simulink model "MotorIdentVel"  (R2013a)
settings: Solver=FixedStepDiscrete  StartTime=0.0  StopTime=Time  FixedStep=0.01  RelTol=1e-3
values from neighbouring files (symbols this model uses):
  joint = CoupledJoints('experiments', 'iCubGenova03', 'torso')    [CoupledExper-IDLE.m]    (also in CoupledExper.m = joint.loadRefFile('ref'); CoupledJoints.m = [joint Motor(date,robotName, part, type,'yaw')]; FrictionTest.m = joint.loadFriction('idle.mat',1); JointStructure.m = struct)
undefined symbols (not defined in the file): Time
libraries: simulink x8, WBCLibrary x7, utility x1
settings Model: Creator=Raffaello  LastModifiedBy=Raffaello
settings DataIOCC: LimitDataPoints=off  OutputSaveName=out

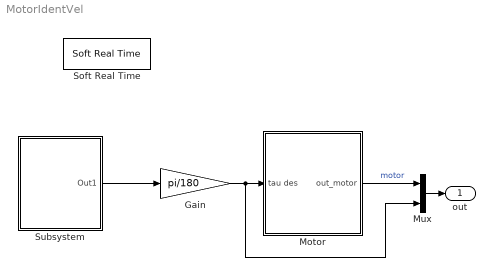
== system MotorIdentVel ==
  Gain : Gain  Gain=pi/180
  Motor : Subsystem
  Mux : Mux  Inputs=2
  Soft Real Time : utility/Soft Real Time  x=1
  Subsystem : Subsystem  mask{time_max=2, time=Time, K=10}
      mask prompts: time_max "Time to max"; K "Max value"
  out : Outport
  wires:
  Motor/1(out_motor) -> Mux/1  "motor"
  Mux/1 -> out/1
  Gain/1 -> Mux/2, Motor/1(tau des)
  Subsystem/1(Out1) -> Gain/1

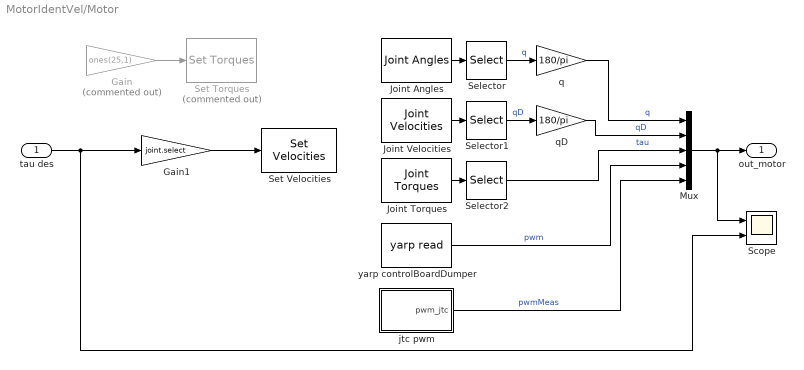
== system MotorIdentVel/Motor ==
  tau des : Inport
  Gain : Gain  Commented=on  Gain=ones(25,1)
  Gain1 : Gain  Gain=joint.select
  Joint Angles : WBCLibrary/wholeBodyStates/Joint Angles  robotName=robotName  localName=localName
  Joint Torques : WBCLibrary/wholeBodyStates/Joint Torques  robotName=robotName  localName=localName
  Joint Velocities : WBCLibrary/wholeBodyStates/Joint Velocities  robotName=robotName  localName=localName
  Mux : Mux  Inputs=5
  Scope : Scope  NumInputPorts=2
      settings: ShowLegends=on  TimeRange=10  YMin=-125~-2  YMax=125~1.5  SaveName=ScopeData2
  Selector : Selector  InputPortWidth=25  IndexOptions=Index vector (dialog)  Indices=[joint.number]  OutputSizes=1
  Selector1 : Selector  InputPortWidth=25  IndexOptions=Index vector (dialog)  Indices=[joint.number]  OutputSizes=1
  Selector2 : Selector  InputPortWidth=25  IndexOptions=Index vector (dialog)  Indices=[joint.number]  OutputSizes=1
  Set Torques : WBCLibrary/wholeBodyActuators/Set Torques  Commented=on  val=6  robotName=robotName  localName=localName
  Set Velocities : WBCLibrary/wholeBodyActuators/Set Velocities  val=4  robotName=robotName  localName=localName
  jtc pwm : Subsystem
  q : Gain  Gain=180/pi
  qD : Gain  Gain=180/pi
  yarp controlBoardDumper : WBCLibrary/Utilities/yarp read  from=['/controlBoardDumper/' joint.path '/getOutputs']  to='...'  num=1  blocking=off  timestamp=off
  out_motor : Outport
  wires:
  Gain/1 -> Set Torques/1
  Joint Velocities/1 -> Selector1/1
  Mux/1 -> out_motor/1, Scope/1
  Joint Angles/1 -> Selector/1
  Joint Torques/1 -> Selector2/1
  yarp controlBoardDumper/1 -> Mux/4  "pwm"
  Selector/1 -> q/1  "q"
  Selector1/1 -> qD/1  "qD"
  Selector2/1 -> Mux/3  "tau"
  q/1 -> Mux/1  "q"
  qD/1 -> Mux/2  "qD"
  jtc pwm/1(pwm_jtc) -> Mux/5  "pwmMeas"
  tau des/1 -> Gain1/1, Scope/2
  Gain1/1 -> Set Velocities/1

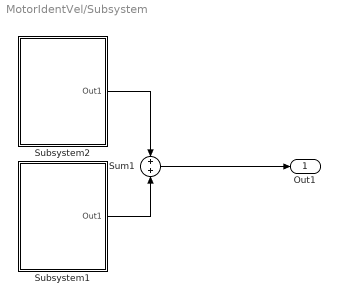
== system MotorIdentVel/Subsystem ==
  Subsystem1 : Subsystem  mask{time_max=time_max, init=0, K=-K, tot_time=time/2, time_start=time/2}
      mask prompts: time_max "Time to max"; init "Initial value"; K "Max value"; tot_time "Total time"; time_start "Time start"
  Subsystem2 : Subsystem  mask{time_max=time_max, init=0, K=K, tot_time=time/2, time_start=0}
      mask prompts: time_max "Time to max"; init "Initial value"; K "Max value"; tot_time "Total time"; time_start "Time start"
  Sum1 : Sum
  Out1 : Outport
  wires:
  Subsystem2/1(Out1) -> Sum1/1
  Subsystem1/1(Out1) -> Sum1/2
  Sum1/1 -> Out1/1

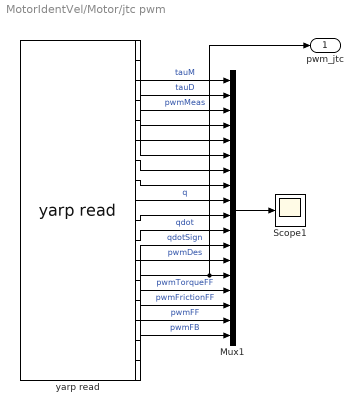
== system MotorIdentVel/Motor/jtc pwm ==
  Mux1 : Mux  Inputs=18
  Scope1 : Scope
      settings: ShowLegends=on
  yarp read : WBCLibrary/Utilities/yarp read  from=['/jtc/monitor:o']  to='...'  num=18  blocking=off  timestamp=off
  pwm_jtc : Outport
  wires:
  yarp read/18 -> Mux1/18  "pwmFB"
  Mux1/1 -> Scope1/1
  yarp read/1 -> Mux1/1  "tauM"
  yarp read/2 -> Mux1/2  "tauD"
  yarp read/3 -> Mux1/3
  yarp read/4 -> Mux1/4
  yarp read/5 -> Mux1/5
  yarp read/10 -> Mux1/10
  yarp read/6 -> Mux1/6
  yarp read/7 -> Mux1/7
  yarp read/8 -> Mux1/8
  yarp read/9 -> Mux1/9  "q"
  yarp read/11 -> Mux1/11  "qdot"
  yarp read/12 -> Mux1/12  "qdotSign"
  yarp read/13 -> Mux1/13  "pwmDes"
  yarp read/14 -> pwm_jtc/1, Mux1/14  "pwmMeas"
  yarp read/15 -> Mux1/15  "pwmTorqueFF"
  yarp read/16 -> Mux1/16  "pwmFrictionFF"
  yarp read/17 -> Mux1/17  "pwmFF"

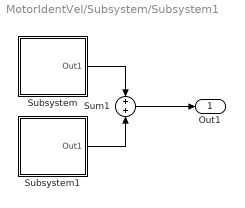
== system MotorIdentVel/Subsystem/Subsystem1 ==
  Subsystem : Subsystem  mask{Start=time_max, K=K, Init=init, time_start=time_start}
      mask prompts: Start "Time to max"; K "Max"; Init "Init value"; time_start "Time Start"
  Subsystem1 : Subsystem  mask{Start=time_max, K=-K, Init=0, time_start=time_start + tot_time - time_max}
      mask prompts: Start "Time to max"; K "Max"; Init "Init value"; time_start "Time Start"
  Sum1 : Sum
  Out1 : Outport
  wires:
  Sum1/1 -> Out1/1
  Subsystem/1(Out1) -> Sum1/1
  Subsystem1/1(Out1) -> Sum1/2

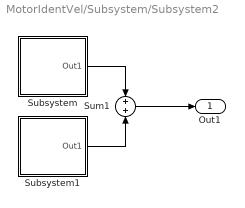
== system MotorIdentVel/Subsystem/Subsystem2 ==
  Subsystem : Subsystem  mask{Start=time_max, K=K, Init=init, time_start=time_start}
      mask prompts: Start "Time to max"; K "Max"; Init "Init value"; time_start "Time Start"
  Subsystem1 : Subsystem  mask{Start=time_max, K=-K, Init=0, time_start=time_start + tot_time - time_max}
      mask prompts: Start "Time to max"; K "Max"; Init "Init value"; time_start "Time Start"
  Sum1 : Sum
  Out1 : Outport
  wires:
  Sum1/1 -> Out1/1
  Subsystem/1(Out1) -> Sum1/1
  Subsystem1/1(Out1) -> Sum1/2

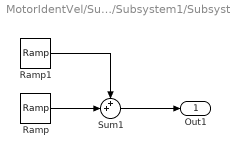
== system MotorIdentVel/Subsystem/Subsystem1/Subsystem ==
  Ramp : simulink/Sources/Ramp  slope=K/Start  start=time_start  X0=Init
  Ramp1 : simulink/Sources/Ramp  slope=-K/Start  start=time_start + Start  X0=0
  Sum1 : Sum  Inputs=++|
  Out1 : Outport
  wires:
  Sum1/1 -> Out1/1
  Ramp/1 -> Sum1/2
  Ramp1/1 -> Sum1/1

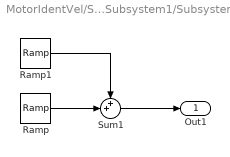
== system MotorIdentVel/Subsystem/Subsystem1/Subsystem1 ==
  Ramp : simulink/Sources/Ramp  slope=K/Start  start=time_start  X0=Init
  Ramp1 : simulink/Sources/Ramp  slope=-K/Start  start=time_start + Start  X0=0
  Sum1 : Sum  Inputs=++|
  Out1 : Outport
  wires:
  Sum1/1 -> Out1/1
  Ramp/1 -> Sum1/2
  Ramp1/1 -> Sum1/1

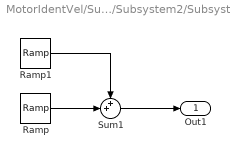
== system MotorIdentVel/Subsystem/Subsystem2/Subsystem ==
  Ramp : simulink/Sources/Ramp  slope=K/Start  start=time_start  X0=Init
  Ramp1 : simulink/Sources/Ramp  slope=-K/Start  start=time_start + Start  X0=0
  Sum1 : Sum  Inputs=++|
  Out1 : Outport
  wires:
  Sum1/1 -> Out1/1
  Ramp/1 -> Sum1/2
  Ramp1/1 -> Sum1/1

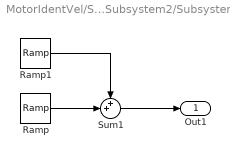
== system MotorIdentVel/Subsystem/Subsystem2/Subsystem1 ==
  Ramp : simulink/Sources/Ramp  slope=K/Start  start=time_start  X0=Init
  Ramp1 : simulink/Sources/Ramp  slope=-K/Start  start=time_start + Start  X0=0
  Sum1 : Sum  Inputs=++|
  Out1 : Outport
  wires:
  Sum1/1 -> Out1/1
  Ramp/1 -> Sum1/2
  Ramp1/1 -> Sum1/1
